simulink library "pwrsys"  (R2018a)
settings: Solver=VariableStepAuto  StartTime=0.0  StopTime=10.0  RelTol=1e-3
values from neighbouring files (symbols this model uses):
  Ts = Ts_c    (= 1e-07)    [PlantStateEquations_abc_Script.m]
undefined symbols (not defined in the file or in its folder): D1, Delta, DiscIntNeverNeededParam, ESS, f_LPF_noise, fn, fsw, grid, gt1, Iap, Kp, PCC, Refmax, Refmin, sim, SIMU, Sn, tctrl, Ti, Ts_control, Ts_PWM, Uabp, Uanp, WT, X, zeta
libraries: $bdroot x71, powerlib x59, powerlib_meascontrol x49, peTransforms x20, PhD_Library x1, sps_avr x1
(part 2 of 4)

== system pwrsys/Basic Blocks/PI_Kg_Kp_Ti_AntiWindup ==
  note: PI: Kg (Kp + 1/sTi)
  error : Inport
  DisableP : Inport  Port=2
  Ihold : Inport  Port=3
  force_int : Inport  Port=4
  force_val : Inport  Port=5
  Add1 : Sum
  Add9 : Sum
  Constant : Constant  Value=PI_max
  Constant1 : Constant  Value=PI_min
  Constant8 : Constant  Value=0
  Gain1 : Gain  Gain=Kp
  Gain7 : Gain  Gain=Kg
  Gain9 : Gain  Gain=1/Ti
  NotEqual : RelationalOperator  Operator=~=  OutDataTypeStr=boolean  RndMeth=Simplest
  Product : Product
  Relay : Relay  OnSwitchValue=0.6  OffSwitchValue=0.4  OnOutputValue=0  OffOutputValue=1
  Saturation1 : Saturate  UpperLimit=PI_max  LowerLimit=PI_min
  Switch : Switch  Criteria=u2 > Threshold
  digital_integrator : $bdroot/Basic Blocks/digital_integrator  Ts=Ts
  out : Outport
  Punlim : Outport  Port=2
  I : Outport  Port=3
  wires:
  NotEqual/1 -> [StopInt]
  Saturation1/1 -> out/1, NotEqual/2
  error/1 -> Gain7/1
  digital_integrator/1 -> I/1, Add9/2
  Add1/1 -> Switch/2
  Constant8/1 -> Switch/1
  Gain7/1 -> Gain1/1, Switch/3
  Switch/1 -> Gain9/1
  Add9/1 -> NotEqual/1, Saturation1/1
  Gain9/1 -> digital_integrator/1
  [StopInt] -> Add1/1
  Ihold/1 -> Add1/2
  Product/1 -> Punlim/1, Add9/1
  Gain1/1 -> Product/2
  DisableP/1 -> Relay/1
  Relay/1 -> Product/1
  force_val/1 -> digital_integrator/5
  force_int/1 -> digital_integrator/4
  Constant1/1 -> digital_integrator/3
  Constant/1 -> digital_integrator/2

== system pwrsys/Basic Blocks/PI_Kp_Ti_AntiWindup ==
  note: PI: Kp (s Ti + 1) / (s Ti)
  error : Inport
  Ihold : Inport  Port=2
  force_int : Inport  Port=3
  force_val : Inport  Port=4
  Add1 : Sum
  Add9 : Sum
  Constant : Constant  Value=PI_max
  Constant1 : Constant  Value=PI_min
  Constant8 : Constant  Value=0
  Gain7 : Gain  Gain=Kp
  Gain9 : Gain  Gain=1/Ti
  NotEqual : RelationalOperator  Operator=~=  OutDataTypeStr=boolean  RndMeth=Simplest
  Saturation1 : Saturate  UpperLimit=PI_max  LowerLimit=PI_min
  Switch : Switch  Criteria=u2 > Threshold
  digital_integrator : $bdroot/Basic Blocks/digital_integrator  Ts=Ts
  out : Outport
  Punlim : Outport  Port=2
  I : Outport  Port=3
  wires:
  NotEqual/1 -> [StopInt]
  Saturation1/1 -> out/1, NotEqual/2
  error/1 -> Gain7/1
  digital_integrator/1 -> I/1, Add9/2
  Add1/1 -> Switch/2
  Constant8/1 -> Switch/1
  Gain7/1 -> Switch/3, Punlim/1, Add9/1
  Switch/1 -> Gain9/1
  Add9/1 -> NotEqual/1, Saturation1/1
  Gain9/1 -> digital_integrator/1
  [StopInt] -> Add1/1
  Ihold/1 -> Add1/2
  Constant1/1 -> digital_integrator/3
  force_int/1 -> digital_integrator/4
  force_val/1 -> digital_integrator/5
  Constant/1 -> digital_integrator/2

== system pwrsys/Basic Blocks/PQVI ==
  note: Akagi 1984 for p and q
      | calc. without zero seq,
      | factor 3/2 compensates for
      | amplitude invariant
      | Clarke transformation
  valphabeta : Inport
  ialphabeta : Inport  Port=2
  Add3 : Sum  Inputs=+-
  Bus Creator : BusCreator  Inputs=4
  Demux1 : Demux  Outputs=2
  Demux4 : Demux  Outputs=2
  Dot Product : DotProduct  InputSameDT=on  OutDataTypeStr=Inherit: Inherit via internal rule
  Gain1 : Gain  Gain=3/2/Sn
  Gain2 : Gain  Gain=3/2/Sn
  Gain3 : Gain  Gain=1/Uanp
  Gain4 : Gain  Gain=1/Iap
  Hypot : Math  Operator=hypot  RndMeth=Zero  SaturateOnIntegerOverflow=on
  Hypot1 : Math  Operator=hypot  RndMeth=Zero  SaturateOnIntegerOverflow=on
  Product3 : Product
  Product4 : Product
  pqvi : Outport
  wires:
  Gain4/1 -> Bus Creator/4  "i"
  Gain1/1 -> Bus Creator/1  "p"
  Gain2/1 -> Bus Creator/2  "q"
  Product4/1 -> Add3/2
  Dot Product/1 -> Gain1/1  "p"
  Hypot1/1 -> Gain4/1  "i"
  Gain3/1 -> Bus Creator/3  "v"
  Demux1/2 -> Hypot1/2, Product4/2
  valphabeta/1 -> Demux4/1, Dot Product/1
  Demux1/1 -> Hypot1/1, Product3/2
  ialphabeta/1 -> Demux1/1, Dot Product/2
  Add3/1 -> Gain2/1  "q"
  Demux4/2 -> Hypot/2, Product3/1
  Product3/1 -> Add3/1
  Hypot/1 -> Gain3/1  "v"
  Demux4/1 -> Hypot/1, Product4/1
  Bus Creator/1 -> pqvi/1

== system pwrsys/Basic Blocks/digital_integrator ==
  x : Inport
  max : Inport  Port=2
  min : Inport  Port=3
  force_if=1 : Inport  Port=4
  force_value : Inport  Port=5
  Constant : Constant  Value=Ts
  MATLAB Function : MATLAB Function  TreatAsAtomicUnit=on  SystemSampleTime=Ts
      settings: RTWSystemCode=Inline
  y : Outport
  wires:
  x/1 -> MATLAB Function/1(x)
  MATLAB Function/1(y) -> y/1
  max/1 -> MATLAB Function/2(max)
  min/1 -> MATLAB Function/3(min)
  force_if=1/1 -> MATLAB Function/4(force)
  force_value/1 -> MATLAB Function/5(forceval)
  Constant/1 -> MATLAB Function/6(Ts)

== system pwrsys/Basic Blocks/digital_ramp_gen ==
  up_if>0 : Inport
  down_if>0 : Inport  Port=2
  rate_pu/s : Inport  Port=3
  max : Inport  Port=4
  min : Inport  Port=5
  force_if=1 : Inport  Port=6
  force_value : Inport  Port=7
  Constant : Constant  Value=Ts
  MATLAB Function : MATLAB Function  TreatAsAtomicUnit=on  SystemSampleTime=Ts
      settings: RTWSystemCode=Inline
  y : Outport
  wires:
  up_if>0/1 -> MATLAB Function/1(up)
  MATLAB Function/1(y) -> y/1
  max/1 -> MATLAB Function/4(max)
  min/1 -> MATLAB Function/5(min)
  force_if=1/1 -> MATLAB Function/6(force)
  force_value/1 -> MATLAB Function/7(forceval)
  Constant/1 -> MATLAB Function/8(Ts)
  down_if>0/1 -> MATLAB Function/2(down)
  rate_pu/s/1 -> MATLAB Function/3(rate)

== system pwrsys/Basic Blocks/pqui_Transd_DSC ==
  Vabc : Inport
  Iabc : Inport  Port=2
  w_pu : Inport  Port=3
  Clarke Transform{,1..3} (4 alike) : peTransforms/Clarke Transform  PowerInvariant=off
  Constant : Constant
  DSC Power 1 : $bdroot/Basic Blocks/DSC Power 
  DSC Power 2 : $bdroot/Basic Blocks/DSC Power 
  Data Type Conversion1 : DataTypeConversion  OutDataTypeStr=int16  RndMeth=Round  SaturateOnIntegerOverflow=on
  Divide : Product  Inputs=*/
  Gain2 : Gain  Gain=4*Ts*fn
  PQVI : $bdroot/Basic Blocks/PQVI  Sn=Sn  Uanp=Uanp  Iap=Iap
  PQVI_Neg : $bdroot/Basic Blocks/PQVI  Sn=Sn  Uanp=Uanp  Iap=Iap
  PQVI_Pos : $bdroot/Basic Blocks/PQVI  Sn=Sn  Uanp=Uanp  Iap=Iap
  Rate Transition1 : RateTransition  OutPortSampleTime=Ts
  Rate Transition2 : RateTransition  InitialCondition=1  OutPortSampleTime=Ts
  Rate Transition5 : RateTransition  OutPortSampleTime=Ts
  Saturation : Saturate  UpperLimit=inf  LowerLimit=0.000001
  Selector{1,4..6} (4 alike) : Selector  InputPortWidth=3  IndexOptions=Index vector (dialog)  Indices=[1 2]  OutputSizes=1
  Selector2 : Selector  InputPortWidth=3  IndexOptions=Index vector (dialog)  Indices=[1 3 2]  OutputSizes=1
  Selector3 : Selector  InputPortWidth=3  IndexOptions=Index vector (dialog)  Indices=[1 3 2]  OutputSizes=1
  pqvi : Outport
  pqvi+ : Outport  Port=2
  pqvi- : Outport  Port=3
  wires:
  Clarke Transform1/1 -> Selector1/1
  Vabc/1 -> Rate Transition1/1
  Clarke Transform/1 -> Selector5/1
  Iabc/1 -> Rate Transition5/1
  Rate Transition1/1 -> Selector2/1, Clarke Transform/1
  Rate Transition5/1 -> Selector3/1, Clarke Transform1/1
  Selector5/1 -> DSC Power 2/1, PQVI/1
  Selector1/1 -> DSC Power 2/2, PQVI/2
  PQVI/1 -> pqvi/1
  Data Type Conversion1/1 -> DSC Power 1/3, DSC Power 2/3
  DSC Power 2/1 -> PQVI_Pos/1
  DSC Power 2/2 -> PQVI_Pos/2
  PQVI_Pos/1 -> pqvi+/1
  Clarke Transform2/1 -> Selector6/1
  Clarke Transform3/1 -> Selector4/1
  Selector2/1 -> Clarke Transform2/1
  Selector3/1 -> Clarke Transform3/1
  Selector6/1 -> DSC Power 1/1
  Selector4/1 -> DSC Power 1/2
  PQVI_Neg/1 -> pqvi-/1
  DSC Power 1/2 -> PQVI_Neg/2
  DSC Power 1/1 -> PQVI_Neg/1
  Saturation/1 -> Divide/2
  Constant/1 -> Divide/1
  Rate Transition2/1 -> Gain2/1
  w_pu/1 -> Rate Transition2/1
  Gain2/1 -> Saturation/1
  Divide/1 -> Data Type Conversion1/1

== system pwrsys/Basic Blocks/pqui_Transd_NoZeroSeq ==
  note: Akagi 1984 for p and q
      | calc. without zero seq,
      | factor 3/2 compensates for
      | amplitude invariant
      | Clarke transformation
  Vabc : Inport
  Iabc : Inport  Port=2
  Add3 : Sum  Inputs=+-
  Clarke Transform : peTransforms/Clarke Transform  PowerInvariant=off
  Clarke Transform1 : peTransforms/Clarke Transform  PowerInvariant=off
  Demux1 : Demux  Outputs=2
  Demux4 : Demux  Outputs=2
  Dot Product : DotProduct  InputSameDT=on  OutDataTypeStr=Inherit: Inherit via internal rule
  Gain1 : Gain  Gain=3/2/Sn
  Gain2 : Gain  Gain=3/2/Sn
  Gain3 : Gain  Gain=1/Uanp
  Gain4 : Gain  Gain=1/Iap
  Hypot : Math  Operator=hypot  RndMeth=Zero  SaturateOnIntegerOverflow=on
  Hypot1 : Math  Operator=hypot  RndMeth=Zero  SaturateOnIntegerOverflow=on
  Product3 : Product
  Product4 : Product
  Selector1 : Selector  InputPortWidth=3  IndexOptions=Index vector (dialog)  Indices=[1 2]  OutputSizes=1
  Selector5 : Selector  InputPortWidth=3  IndexOptions=Index vector (dialog)  Indices=[1 2]  OutputSizes=1
  p : Outport
  q : Outport  Port=2
  v : Outport  Port=3
  i : Outport  Port=4
  wires:
  Clarke Transform1/1 -> Selector1/1
  Gain3/1 -> v/1  "v"
  Demux1/2 -> Hypot1/2, Product4/2
  Hypot1/1 -> Gain4/1  "i"
  Selector1/1 -> Demux1/1, Dot Product/2
  Selector5/1 -> Demux4/1, Dot Product/1
  Demux4/1 -> Hypot/1, Product4/1
  Hypot/1 -> Gain3/1  "v"
  Dot Product/1 -> Gain1/1  "p"
  Demux1/1 -> Hypot1/1, Product3/2
  Add3/1 -> Gain2/1  "q"
  Product4/1 -> Add3/2
  Demux4/2 -> Hypot/2, Product3/1
  Vabc/1 -> Clarke Transform/1
  Clarke Transform/1 -> Selector5/1
  Iabc/1 -> Clarke Transform1/1
  Product3/1 -> Add3/1
  Gain1/1 -> p/1  "p"
  Gain4/1 -> i/1  "i"
  Gain2/1 -> q/1  "q"

== system pwrsys/Basic Blocks/pqui_Transd_NoZeroSeq_Filter ==
  note: Akagi 1984 for p and q
      | calc. without zero seq,
      | factor 3/2 compensates for
      | amplitude invariant
      | Clarke transformation
  Vabc : Inport
  Iabc : Inport  Port=2
  Add3 : Sum  Inputs=+-
  Clarke Transform : peTransforms/Clarke Transform  PowerInvariant=off
  Clarke Transform1 : peTransforms/Clarke Transform  PowerInvariant=off
  Demux1 : Demux  Outputs=2
  Demux4 : Demux  Outputs=2
  Dot Product : DotProduct  InputSameDT=on  OutDataTypeStr=Inherit: Inherit via internal rule
  Gain1 : Gain  Gain=3/2/Sn
  Gain2 : Gain  Gain=3/2/Sn
  Gain3 : Gain  Gain=1/Uanp
  Gain4 : Gain  Gain=1/Iap
  Hypot : Math  Operator=hypot  RndMeth=Zero  SaturateOnIntegerOverflow=on
  Hypot1 : Math  Operator=hypot  RndMeth=Zero  SaturateOnIntegerOverflow=on
  Product3 : Product
  Product4 : Product
  Rate Transition1 : RateTransition  OutPortSampleTime=Ts
  Rate Transition2 : RateTransition  OutPortSampleTime=Ts
  Second-Order Filter1 : powerlib_meascontrol/Filters/Second-Order Filter  FilterType=Lowpass  Fo=fcutoutvi  Zeta=zeta  Ts=Ts  Initialize=off  Vac_Init="[0,  0,  60]"  Vdc_Init=0  PlotResponse=off  FreqRange=[0, 1000, 0.1]
      settings: SourceProductName=Simscape Power Systems  SourceProductBaseCode=PS
  Second-Order Filter2 : powerlib_meascontrol/Filters/Second-Order Filter  FilterType=Lowpass  Fo=fcutoutvi  Zeta=zeta  Ts=Ts  Initialize=off  Vac_Init="[0,  0,  60]"  Vdc_Init=0  PlotResponse=off  FreqRange=[0, 1000, 0.1]
      settings: SourceProductName=Simscape Power Systems  SourceProductBaseCode=PS
  Second-Order Filter{3,5..6,8} (4 alike) : powerlib_meascontrol/Filters/Second-Order Filter  FilterType=Bandstop (Notch)  Fo=fn  Zeta=zeta  Ts=Ts  Initialize=off  Vac_Init="[0,  0,  60]"  Vdc_Init=0  PlotResponse=off  FreqRange=[0, 1000, 0.1]
      settings: SourceProductName=Simscape Power Systems  SourceProductBaseCode=PS
  Second-Order Filter4 : powerlib_meascontrol/Filters/Second-Order Filter  FilterType=Lowpass  Fo=fcutoutpq  Zeta=zeta  Ts=Ts  Initialize=off  Vac_Init="[0,  0,  60]"  Vdc_Init=0  PlotResponse=off  FreqRange=[0, 1000, 0.1]
      settings: SourceProductName=Simscape Power Systems  SourceProductBaseCode=PS
  Second-Order Filter7 : powerlib_meascontrol/Filters/Second-Order Filter  FilterType=Lowpass  Fo=fcutoutpq  Zeta=zeta  Ts=Ts  Initialize=off  Vac_Init="[0,  0,  60]"  Vdc_Init=0  PlotResponse=off  FreqRange=[0, 1000, 0.1]
      settings: SourceProductName=Simscape Power Systems  SourceProductBaseCode=PS
  Selector1 : Selector  InputPortWidth=3  IndexOptions=Index vector (dialog)  Indices=[1 2]  OutputSizes=1
  Selector5 : Selector  InputPortWidth=3  IndexOptions=Index vector (dialog)  Indices=[1 2]  OutputSizes=1
  p : Outport
  q : Outport  Port=2
  v : Outport  Port=3
  i : Outport  Port=4
  wires:
  Clarke Transform1/1 -> Selector1/1
  Gain3/1 -> Second-Order Filter2/1  "v"
  Demux1/2 -> Hypot1/2, Product4/2
  Hypot1/1 -> Gain4/1  "i"
  Selector1/1 -> Demux1/1, Dot Product/2
  Selector5/1 -> Demux4/1, Dot Product/1
  Demux4/1 -> Hypot/1, Product4/1
  Hypot/1 -> Gain3/1  "v"
  Iabc/1 -> Rate Transition2/1
  Dot Product/1 -> Gain1/1  "p"
  Demux1/1 -> Hypot1/1, Product3/2
  Add3/1 -> Gain2/1  "q"
  Vabc/1 -> Rate Transition1/1
  Product4/1 -> Add3/2
  Demux4/2 -> Hypot/2, Product3/1
  Rate Transition1/1 -> Clarke Transform/1
  Clarke Transform/1 -> Selector5/1
  Rate Transition2/1 -> Clarke Transform1/1
  Product3/1 -> Add3/1
  Gain1/1 -> Second-Order Filter7/1  "p"
  Gain4/1 -> Second-Order Filter1/1  "i"
  Gain2/1 -> Second-Order Filter4/1  "q"
  Second-Order Filter2/1 -> Second-Order Filter5/1
  Second-Order Filter5/1 -> v/1
  Second-Order Filter1/1 -> Second-Order Filter3/1
  Second-Order Filter3/1 -> i/1
  Second-Order Filter4/1 -> Second-Order Filter6/1
  Second-Order Filter6/1 -> q/1
  Second-Order Filter8/1 -> p/1
  Second-Order Filter7/1 -> Second-Order Filter8/1

== system pwrsys/PLLs/PLL ==
  vabc : Inport
  PLL (3ph) : powerlib_meascontrol/PLL/PLL (3ph)  Fmin=0.8*fn  Par_Init=[PLL_ini, fn]  ParK=[Kp_pll, Ki_pll, Kd_pll]  TcD=1e-4  MaxRateChangeFreq=fn/5  FilterCutOffFreq=fn/2  Ts=Ts  AGC=on
  Rate Transition1 : RateTransition  OutPortSampleTime=Ts
  Rtot_pu1 : Gain  Gain=-1  SaturateOnIntegerOverflow=on  OutDataTypeStr=Inherit: Same as input  ParamDataTypeStr=Inherit: Same as input
  Rtot_pu3 : Gain  Gain=1/fn  SaturateOnIntegerOverflow=on  OutDataTypeStr=Inherit: Same as input  ParamDataTypeStr=Inherit: Same as input
  f_pu : Outport
  wt : Outport  Port=2
  minus_wt : Outport  Port=3
  wires:
  Rtot_pu3/1 -> f_pu/1
  vabc/1 -> Rate Transition1/1
  Rate Transition1/1 -> PLL (3ph)/1
  PLL (3ph)/2 -> Rtot_pu1/1, wt/1
  PLL (3ph)/1 -> Rtot_pu3/1
  Rtot_pu1/1 -> minus_wt/1

== system pwrsys/PLLs/PLL 3-phase abc ==
  Vabc : Inport
  120deg : Constant  Value=2/3*pi
  Anti-windup : RelationalOperator  Operator=~=  OutDataTypeStr=boolean  RndMeth=Simplest
  Derivative : Gain  Gain=Kd/Tr
  Discrete-Time Integrator : DiscreteIntegrator  gainval=1/Tr  SampleTime=-1  LimitOutput=on  UpperSaturationLimit=2*pi*fdev  LowerSaturationLimit=-2*pi*fdev  ICPrevOutput=DiscIntNeverNeededParam  ICPrevScaledInput=DiscIntNeverNeededParam
  Dot Product : DotProduct  InputSameDT=on  OutDataTypeStr=Inherit: Inherit via internal rule
  Integrator : Integrator  InitialCondition=wt0  UpperSaturationLimit=1  LowerSaturationLimit=-1  ZeroCross=off
  Mux : Mux  Inputs=2
  Mux1 : Mux  Inputs=3
  PI controller with Hold : $bdroot/Basic Blocks/PI controller  with Hold  Kp=Kp  Ki=Ki  Max=2*pi*fdev  Min=-2*pi*fdev  x0=0  Ts=Ts
  Saturation : Saturate  UpperLimit=2*pi*fdev  LowerLimit=-2*pi*fdev
  Second-Order Filter : powerlib_meascontrol/Filters/Second-Order Filter  FilterType=Lowpass  Fo=wn  Zeta=zeta  Ts=0  Initialize=on  Vac_Init="[0,  0,  60]"  Vdc_Init=2*pi*fnom  PlotResponse=off  FreqRange=[0, 500, 1]
      settings: SourceProductName=Simscape Power Systems  SourceProductBaseCode=PS
  Sum1 : Sum
  Sum2 : Sum  Inputs=+-
  Sum3 : Sum
  Sum4 : Sum  Inputs=+-
  Sum6 : Sum  Inputs=-+
  Trigonometric Function : Trigonometry  Operator=sincos  ApproximationMethod=CORDIC
  Trigonometric Function1 : Trigonometry  ApproximationMethod=CORDIC
  Wrap to pi : MATLABFcn  MATLABFcn=wrapToPi
  w rated : Constant  Value=2*pi*fnom
  w : Outport
  wt : Outport  Port=2
  scwt : Outport  Port=3
  wires:
  Discrete-Time Integrator/1 -> Sum6/1
  Sum6/1 -> Discrete-Time Integrator/1, Sum2/2  "d"
  Derivative/1 -> Sum6/2
  Saturation/1 -> Sum1/1, Anti-windup/2  "dw"
  w rated/1 -> Sum1/2
  Sum1/1 -> Second-Order Filter/1, Integrator/1  "w"
  Integrator/1 -> Wrap to pi/1  "wt"
  Vabc/1 -> Dot Product/1
  PI controller with Hold/1 -> Sum2/1  "pi"
  Sum2/1 -> Anti-windup/1, Saturation/1
  Wrap to pi/1 -> Mux1/1, Trigonometric Function/1, Sum4/1, Sum3/1, wt/1  "wtWrap"
  Trigonometric Function/1 -> Mux/1
  Trigonometric Function/2 -> Mux/2
  Mux/1 -> scwt/1
  120deg/1 -> Sum4/2, Sum3/2
  Sum4/1 -> Mux1/2
  Sum3/1 -> Mux1/3
  Mux1/1 -> Trigonometric Function1/1
  Trigonometric Function1/1 -> Dot Product/2
  Second-Order Filter/1 -> w/1
  Dot Product/1 -> Derivative/1, PI controller with Hold/2
  Anti-windup/1 -> PI controller with Hold/1

== system pwrsys/PLLs/PLL_pu ==
  vabc : Inport
  PLL (3ph) : powerlib_meascontrol/PLL/PLL (3ph)  Fmin=0.8*fn  Par_Init=[PLL_ini, fn]  ParK=[Kp_pll, Ki_pll, Kd_pll]  TcD=1e-4  MaxRateChangeFreq=fn/5  FilterCutOffFreq=fn/2  Ts=Ts  AGC=on
  Rate Transition1 : RateTransition  OutPortSampleTime=Ts
  Rtot_pu3 : Gain  Gain=1/fn  SaturateOnIntegerOverflow=on  OutDataTypeStr=Inherit: Same as input  ParamDataTypeStr=Inherit: Same as input
  wt : Outport
  f_pu : Outport  Port=2
  wires:
  Rtot_pu3/1 -> f_pu/1
  vabc/1 -> Rate Transition1/1
  Rate Transition1/1 -> PLL (3ph)/1
  PLL (3ph)/2 -> wt/1
  PLL (3ph)/1 -> Rtot_pu3/1

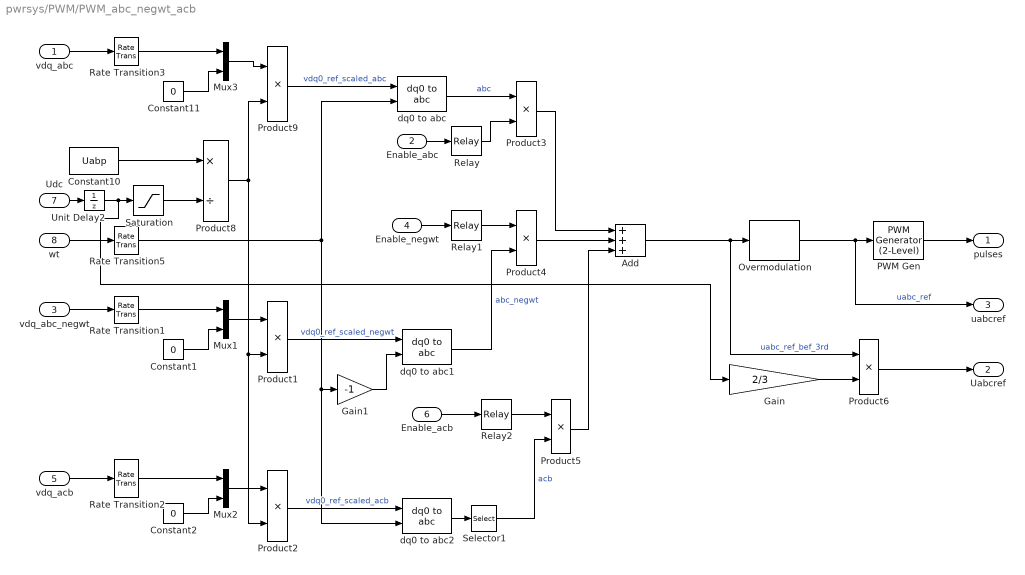
== system pwrsys/PWM/PWM_abc_negwt_acb ==
  vdq_abc : Inport
  Enable_abc : Inport  Port=2
  vdq_abc_negwt : Inport  Port=3
  Enable_negwt : Inport  Port=4
  vdq_acb : Inport  Port=5
  Enable_acb : Inport  Port=6
  Udc : Inport  Port=7
  wt : Inport  Port=8
  Add : Sum  Inputs=+++
  Constant1 : Constant  Value=0
  Constant10 : Constant  Value=Uabp
  Constant11 : Constant  Value=0
  Constant2 : Constant  Value=0
  Gain : Gain  Gain=2/3
  Gain1 : Gain  Gain=-1
  Mux1 : Mux  Inputs=[2 1]
  Mux2 : Mux  Inputs=[2 1]
  Mux3 : Mux  Inputs=[2 1]
  Overmodulation : powerlib_meascontrol/Pulse & Signal Generators/Overmodulation  OverModType=Third harmonic
      settings: SourceProductName=Simscape Power Systems  SourceProductBaseCode=PS
  PWM Gen : powerlib_meascontrol/Pulse & Signal Generators/PWM Generator (2-Level)  ModulatorType=Three-phase bridge (6 pulses)  ModulatorMode=Unsynchronized  Fc=fsw  Pc=PWM_Ini_Phase  nF=27  MinMax="[ -1  1 ]"  SamplingTechnique=Asymmetrical regular (double edge)  ModulatingSignals=off  m=0.8  Freq=60  Phase=0  Ts=Ts  ShowCarrierOutport=off
      settings: SourceProductName=Simscape Power Systems
  Product{1..6,9} (7 alike) : Product  Inputs=**
  Product8 : Product  Inputs=*/
  Rate Transition{1..3,5} (4 alike) : RateTransition  OutPortSampleTime=Ts
  Relay : Relay  OnSwitchValue=0.6  OffSwitchValue=0.4
  Relay1 : Relay  OnSwitchValue=0.6  OffSwitchValue=0.4
  Relay2 : Relay  OnSwitchValue=0.6  OffSwitchValue=0.4
  Saturation : Saturate  UpperLimit=10*Uabp  LowerLimit=0.001*Uabp
  Selector1 : Selector  InputPortWidth=3  IndexOptions=Index vector (dialog)  Indices=[1 3 2]  OutputSizes=1
  Unit Delay2 : UnitDelay  InitialCondition=Uabp  SampleTime=Ts
  dq0 to abc : powerlib_meascontrol/Transformations/dq0 to abc  Alignment=90 degrees behind phase A axis
  dq0 to abc1 : powerlib_meascontrol/Transformations/dq0 to abc  Alignment=90 degrees behind phase A axis
  dq0 to abc2 : powerlib_meascontrol/Transformations/dq0 to abc  Alignment=90 degrees behind phase A axis
  pulses : Outport
  Uabcref : Outport  Port=2
  uabcref : Outport  Port=3
  wires:
  dq0 to abc1/1 -> Product4/2  "abc_negwt"
  Gain1/1 -> dq0 to abc1/2
  Product1/1 -> dq0 to abc1/1  "vdq0_ref_scaled_negwt"
  vdq_abc_negwt/1 -> Rate Transition1/1
  Constant1/1 -> Mux1/2
  Mux1/1 -> Product1/1
  Rate Transition1/1 -> Mux1/1
  Product6/1 -> Uabcref/1
  vdq_abc/1 -> Rate Transition3/1
  PWM Gen/1 -> pulses/1
  Udc/1 -> Unit Delay2/1
  Overmodulation/1 -> uabcref/1, PWM Gen/1  "uabc_ref"
  Constant10/1 -> Product8/1
  wt/1 -> Rate Transition5/1
  Rate Transition3/1 -> Mux3/1
  Mux3/1 -> Product9/1
  Unit Delay2/1 -> Gain/1, Saturation/1
  Product9/1 -> dq0 to abc/1  "vdq0_ref_scaled_abc"
  Rate Transition5/1 -> dq0 to abc/2, dq0 to abc2/2, Gain1/1
  Constant11/1 -> Mux3/2
  dq0 to abc/1 -> Product3/1  "abc"
  Enable_abc/1 -> Relay/1
  Enable_negwt/1 -> Relay1/1
  Add/1 -> Product6/1, Overmodulation/1  "uabc_ref_bef_3rd"
  Saturation/1 -> Product8/2
  Product8/1 -> Product2/2, Product1/2, Product9/2
  Rate Transition2/1 -> Mux2/1
  vdq_acb/1 -> Rate Transition2/1
  Enable_acb/1 -> Relay2/1
  Mux2/1 -> Product2/1
  Constant2/1 -> Mux2/2
  Product2/1 -> dq0 to abc2/1  "vdq0_ref_scaled_acb"
  dq0 to abc2/1 -> Selector1/1
  Selector1/1 -> Product5/2  "acb"
  Relay/1 -> Product3/2
  Product3/1 -> Add/1
  Product4/1 -> Add/2
  Relay1/1 -> Product4/1
  Relay2/1 -> Product5/1
  Product5/1 -> Add/3
  Gain/1 -> Product6/2

== system pwrsys/PWM/PWM_single_dual ==
  vdq_single : Inport
  Enable_single : Inport  Port=2
  vdq_dual_pos : Inport  Port=3
  vdq_dual_neg : Inport  Port=4
  Enable_dual : Inport  Port=5
  Udc : Inport  Port=6
  wt : Inport  Port=7
  Add : Sum  Inputs=+++
  Constant1 : Constant  Value=0
  Constant10 : Constant  Value=Uabp
  Constant11 : Constant  Value=0
  Constant2 : Constant  Value=0
  Gain : Gain  Gain=2/3
  Mux1 : Mux  Inputs=[2 1]
  Mux2 : Mux  Inputs=[2 1]
  Mux3 : Mux  Inputs=[2 1]
  Overmodulation : powerlib_meascontrol/Pulse & Signal Generators/Overmodulation  OverModType=Third harmonic
      settings: SourceProductName=Simscape Power Systems  SourceProductBaseCode=PS
  PWM Gen : powerlib_meascontrol/Pulse & Signal Generators/PWM Generator (2-Level)  ModulatorType=Three-phase bridge (6 pulses)  ModulatorMode=Unsynchronized  Fc=fsw  Pc=PWM_Ini_Phase  nF=27  MinMax="[ -1  1 ]"  SamplingTechnique=Asymmetrical regular (double edge)  ModulatingSignals=off  m=0.8  Freq=60  Phase=0  Ts=Ts  ShowCarrierOutport=off
      settings: SourceProductName=Simscape Power Systems
  Product{1..6,9} (7 alike) : Product  Inputs=**
  Product8 : Product  Inputs=*/
  Rate Transition{1..3,5} (4 alike) : RateTransition  OutPortSampleTime=Ts
  Relay : Relay  OnSwitchValue=0.6  OffSwitchValue=0.4
  Relay1 : Relay  OnSwitchValue=0.6  OffSwitchValue=0.4
  Saturation : Saturate  UpperLimit=10*Uabp  LowerLimit=0.001*Uabp
  Selector1 : Selector  InputPortWidth=3  IndexOptions=Index vector (dialog)  Indices=[1 3 2]  OutputSizes=1
  Unit Delay2 : UnitDelay  InitialCondition=Uabp  SampleTime=Ts
  dq0 to abc : powerlib_meascontrol/Transformations/dq0 to abc  Alignment=90 degrees behind phase A axis
  dq0 to abc1 : powerlib_meascontrol/Transformations/dq0 to abc  Alignment=90 degrees behind phase A axis
  dq0 to abc2 : powerlib_meascontrol/Transformations/dq0 to abc  Alignment=90 degrees behind phase A axis
  pulses : Outport
  Uabcref : Outport  Port=2
  uabcref : Outport  Port=3
  wires:
  dq0 to abc1/1 -> Product4/2  "abc_ref_dual_pos"
  Rate Transition5/1 -> dq0 to abc/2, dq0 to abc1/2, dq0 to abc2/2
  Product1/1 -> dq0 to abc1/1  "vdq0_ref_scaled_dual_pos"
  vdq_dual_pos/1 -> Rate Transition1/1
  Constant1/1 -> Mux1/2
  Mux1/1 -> Product1/1
  Rate Transition1/1 -> Mux1/1
  Product6/1 -> Uabcref/1
  vdq_single/1 -> Rate Transition3/1
  PWM Gen/1 -> pulses/1
  Udc/1 -> Unit Delay2/1
  Overmodulation/1 -> uabcref/1, PWM Gen/1  "uabc_ref"
  Constant10/1 -> Product8/1
  wt/1 -> Rate Transition5/1
  Rate Transition3/1 -> Mux3/1
  Mux3/1 -> Product9/1
  Unit Delay2/1 -> Gain/1, Saturation/1
  Product9/1 -> dq0 to abc/1  "vdq0_ref_scaled_single"
  Constant11/1 -> Mux3/2
  dq0 to abc/1 -> Product3/1  "abc_ref_single"
  Enable_single/1 -> Relay/1
  Enable_dual/1 -> Relay1/1
  Add/1 -> Product6/1, Overmodulation/1  "uabc_ref_bef_3rd"
  Saturation/1 -> Product8/2
  Product8/1 -> Product2/2, Product1/2, Product9/2
  Rate Transition2/1 -> Mux2/1
  vdq_dual_neg/1 -> Rate Transition2/1
  Mux2/1 -> Product2/1
  Constant2/1 -> Mux2/2
  Product2/1 -> dq0 to abc2/1  "vdq0_ref_scaled_dual_neg"
  dq0 to abc2/1 -> Selector1/1
  Selector1/1 -> Product5/2  "abc_ref_dual_neg"
  Relay/1 -> Product3/2
  Product3/1 -> Add/1
  Product4/1 -> Add/2
  Relay1/1 -> Product5/1, Product4/1
  Product5/1 -> Add/3
  Gain/1 -> Product6/2

== system pwrsys/Power Theories/Instantaneous Power xyz ==
  Vxyz : Inport
  Ixyz : Inport  Port=2
  Constant1 : Constant  Value=[a 0 0; 0 a 0; 0 0 b]
  Cross product terms : Product  RndMeth=Zero
  Demux2 : Demux  Outputs=2
  Dot Product : DotProduct  InputSameDT=on  OutDataTypeStr=Inherit: Inherit via internal rule
  Dot Product1 : DotProduct  InputSameDT=on  OutDataTypeStr=Inherit: Inherit via internal rule
  I elements : Selector  InputPortWidth=3  IndexOptions=Index vector (dialog)  Indices=[3 1 2 2 3 1]  OutputSizes=1
  P0 mult : Product  RndMeth=Zero
  Product3 : Product  Multiplication=Matrix(*)
  Q calc : Sum  Inputs=+-
  Sqrt : Sqrt  SaturateOnIntegerOverflow=on
  V elements : Selector  InputPortWidth=3  IndexOptions=Index vector (dialog)  Indices=[2 3 1 3 1 2]  OutputSizes=1
  i0 : Selector  InputPortWidth=3  IndexOptions=Index vector (dialog)  Indices=[3]  OutputSizes=1
  v0 : Selector  InputPortWidth=3  IndexOptions=Index vector (dialog)  Indices=[3]  OutputSizes=1
  P : Outport
  P0 : Outport  Port=2
  Qmat : Outport  Port=3
  Qnorm : Outport  Port=4
  wires:
  Dot Product/1 -> P/1  "P"
  Q calc/1 -> Qmat/1, Dot Product1/2, Dot Product1/1  "Qmat"
  Constant1/1 -> Product3/1
  Product3/1 -> V elements/1, v0/1, Dot Product/1
  Demux2/1 -> Q calc/1
  I elements/1 -> Cross product terms/2
  Vxyz/1 -> Product3/2
  Demux2/2 -> Q calc/2
  Ixyz/1 -> I elements/1, i0/1, Dot Product/2
  V elements/1 -> Cross product terms/1
  Cross product terms/1 -> Demux2/1
  v0/1 -> P0 mult/1
  i0/1 -> P0 mult/2
  P0 mult/1 -> P0/1  "P0"
  Dot Product1/1 -> Sqrt/1
  Sqrt/1 -> Qnorm/1  "Qnorm"

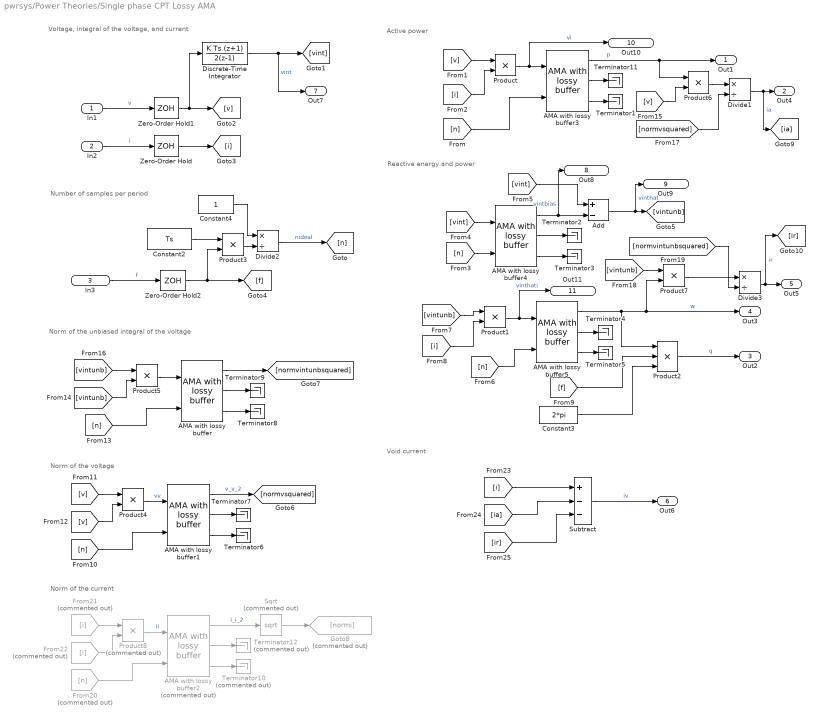
== system pwrsys/Power Theories/Single phase CPT Lossy AMA ==
  note: Voltage, integral of the voltage, and current
  note: Number of samples per period
  note: Norm of the unbiased integral of the voltage
  note: Norm of the voltage
  note: Active power
  note: Reactive energy and power
  note: Norm of the current
  note: Void current
  In1 : Inport
  In2 : Inport  Port=2
  In3 : Inport  Port=3
  AMA with lossy buffer{,1,3..5} (5 alike) : $bdroot/Adaptive Moving Averages/AMA with lossy buffer  NbSize=NbSize  Ts=Ts
  AMA with lossy buffer2 : $bdroot/Adaptive Moving Averages/AMA with lossy buffer  Commented=on  NbSize=NbSize  Ts=Ts
  Add : Sum  Inputs=+-
  Constant2 : Constant  Value=Ts
  Constant3 : Constant  Value=2*pi
  Constant4 : Constant
  Discrete-Time Integrator : DiscreteIntegrator  IntegratorMethod=Integration: Trapezoidal  SampleTime=Ts  ICPrevOutput=DiscIntNeverNeededParam  ICPrevScaledInput=DiscIntNeverNeededParam
  Divide1 : Product  Inputs=*/
  Divide2 : Product  Inputs=*/
  Divide3 : Product  Inputs=*/
  From20 : From  Commented=on  GotoTag=n
  From21 : From  Commented=on  GotoTag=i
  From22 : From  Commented=on  GotoTag=i
  Goto8 : Goto  Commented=on  GotoTag=normi
  Product{,1,3..7} (7 alike) : Product
  Product2 : Product  Inputs=3
  Product8 : Product  Commented=on
  Sqrt : Sqrt  Commented=on  SaturateOnIntegerOverflow=on
  Subtract : Sum  Inputs=+--
  Terminator{1..9,11} (10 alike) : Terminator
  Terminator10 : Terminator  Commented=on
  Terminator12 : Terminator  Commented=on
  Zero-Order Hold : ZeroOrderHold  SampleTime=Ts
  Zero-Order Hold1 : ZeroOrderHold  SampleTime=Ts
  Zero-Order Hold2 : ZeroOrderHold  SampleTime=Ts
  Out1 : Outport
  Out4 : Outport  Port=2
  Out2 : Outport  Port=3
  Out3 : Outport  Port=4
  Out5 : Outport  Port=5
  Out6 : Outport  Port=6
  Out7 : Outport  Port=7
  Out8 : Outport  Port=8
  Out9 : Outport  Port=9
  Out10 : Outport  Port=10
  Out11 : Outport  Port=11
  wires:
  [n] -> AMA with lossy buffer3/2
  AMA with lossy buffer3/2 -> Terminator11/1
  AMA with lossy buffer3/3 -> Terminator1/1
  Product1/1 -> Out11/1, AMA with lossy buffer5/1  "vinthati"
  AMA with lossy buffer4/1 -> Out8/1, Add/2  "vintbias"
  AMA with lossy buffer4/2 -> Terminator2/1
  [n] -> AMA with lossy buffer4/2
  AMA with lossy buffer5/3 -> Terminator5/1
  AMA with lossy buffer4/3 -> Terminator3/1
  [n] -> AMA with lossy buffer5/2
  AMA with lossy buffer5/1 -> Product7/2, Out3/1, Product2/1  "w"
  [i] -> Product/2
  In1/1 -> Zero-Order Hold1/1  "v"
  In2/1 -> Zero-Order Hold/1  "i"
  [vint] -> Add/1
  Constant4/1 -> Divide2/1
  Divide2/1 -> [n]  "nideal"
  Product3/1 -> Divide2/2
  [v] -> Product/1
  Constant2/1 -> Product3/1
  AMA with lossy buffer5/2 -> Terminator4/1
  [f] -> Product2/2
  Constant3/1 -> Product2/3
  [i] -> Product1/2
  [vint] -> AMA with lossy buffer4/1
  Zero-Order Hold1/1 -> [v], Discrete-Time Integrator/1
  AMA with lossy buffer3/1 -> Product6/1, Out1/1  "p"
  [vintunb] -> Product1/1
  In3/1 -> Zero-Order Hold2/1  "f"
  Product/1 -> Out10/1, AMA with lossy buffer3/1  "vi"
  Zero-Order Hold2/1 -> Product3/2, [f]
  Zero-Order Hold/1 -> [i]
  Product2/1 -> Out2/1  "q"
  Discrete-Time Integrator/1 -> Out7/1, [vint]  "vint"
  Add/1 -> Out9/1, [vintunb]  "vinthat"
  AMA with lossy buffer1/3 -> Terminator6/1
  AMA with lossy buffer1/2 -> Terminator7/1
  AMA with lossy buffer1/1 -> [normvsquared]  "v_v_2"
  [v] -> Product4/1
  [n] -> AMA with lossy buffer1/2
  Product4/1 -> AMA with lossy buffer1/1  "vv"
  [v] -> Product4/2
  [n] -> AMA with lossy buffer/2
  AMA with lossy buffer/2 -> Terminator9/1
  AMA with lossy buffer/1 -> [normvintunbsquared]
  [vintunb] -> Product5/1
  Product5/1 -> AMA with lossy buffer/1
  AMA with lossy buffer/3 -> Terminator8/1
  [vintunb] -> Product5/2
  [v] -> Product6/2
  Product6/1 -> Divide1/1
  [normvsquared] -> Divide1/2
  Divide1/1 -> [ia], Out4/1  "ia"
  [vintunb] -> Product7/1
  Product7/1 -> Divide3/1
  [normvintunbsquared] -> Divide3/2
  Divide3/1 -> [ir], Out5/1  "ir"
  From20/1 -> AMA with lossy buffer2/2
  AMA with lossy buffer2/2 -> Terminator12/1
  AMA with lossy buffer2/1 -> Sqrt/1  "i_i_2"
  From21/1 -> Product8/1
  Product8/1 -> AMA with lossy buffer2/1  "ii"
  AMA with lossy buffer2/3 -> Terminator10/1
  From22/1 -> Product8/2
  Sqrt/1 -> Goto8/1
  [i] -> Subtract/1
  [ia] -> Subtract/2
  [ir] -> Subtract/3
  Subtract/1 -> Out6/1  "iv"

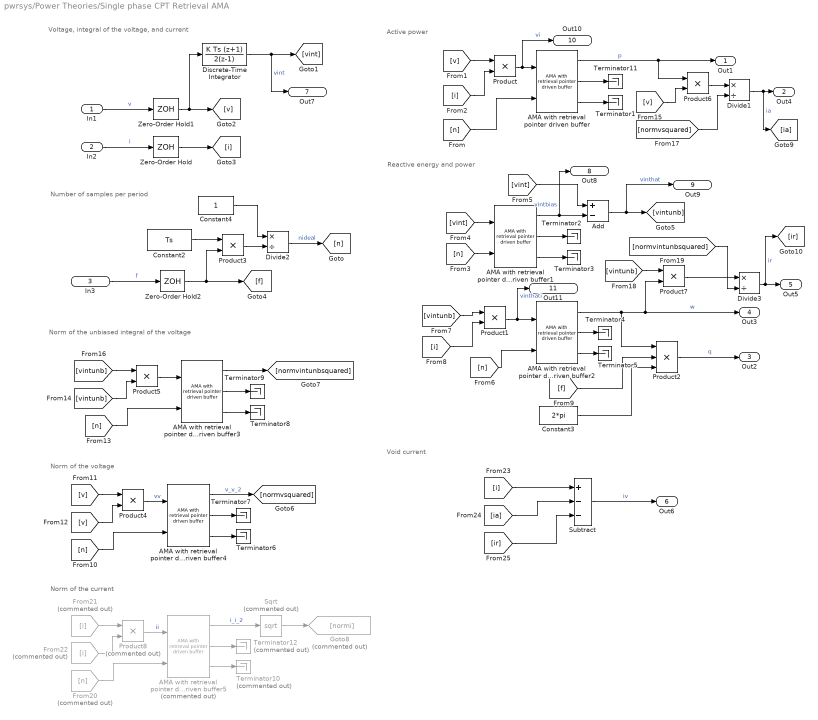
== system pwrsys/Power Theories/Single phase CPT Retrieval AMA ==
  note: Norm of the voltage
  note: Void current
  note: Active power
  note: Norm of the current
  note: Number of samples per period
  note: Norm of the unbiased integral of the voltage
  note: Reactive energy and power
  note: Voltage, integral of the voltage, and current
  In1 : Inport
  In2 : Inport  Port=2
  In3 : Inport  Port=3
  AMA with retrieval pointer driven buffer{,1..4} (5 alike) : $bdroot/Adaptive Moving Averages/AMA with retrieval pointer driven buffer  NbSize=NbSize  Ts=Ts
  AMA with retrieval pointer driven buffer5 : $bdroot/Adaptive Moving Averages/AMA with retrieval pointer driven buffer  Commented=on  NbSize=NbSize  Ts=Ts
  Add : Sum  Inputs=+-
  Constant2 : Constant  Value=Ts
  Constant3 : Constant  Value=2*pi
  Constant4 : Constant
  Discrete-Time Integrator : DiscreteIntegrator  IntegratorMethod=Integration: Trapezoidal  SampleTime=Ts  ICPrevOutput=DiscIntNeverNeededParam  ICPrevScaledInput=DiscIntNeverNeededParam
  Divide1 : Product  Inputs=*/
  Divide2 : Product  Inputs=*/
  Divide3 : Product  Inputs=*/
  From20 : From  Commented=on  GotoTag=n
  From21 : From  Commented=on  GotoTag=i
  From22 : From  Commented=on  GotoTag=i
  Goto8 : Goto  Commented=on  GotoTag=normi
  Product{,1,3..7} (7 alike) : Product
  Product2 : Product  Inputs=3
  Product8 : Product  Commented=on
  Sqrt : Sqrt  Commented=on  SaturateOnIntegerOverflow=on
  Subtract : Sum  Inputs=+--
  Terminator{1..9,11} (10 alike) : Terminator
  Terminator10 : Terminator  Commented=on
  Terminator12 : Terminator  Commented=on
  Zero-Order Hold : ZeroOrderHold  SampleTime=Ts
  Zero-Order Hold1 : ZeroOrderHold  SampleTime=Ts
  Zero-Order Hold2 : ZeroOrderHold  SampleTime=Ts
  Out1 : Outport
  Out4 : Outport  Port=2
  Out2 : Outport  Port=3
  Out3 : Outport  Port=4
  Out5 : Outport  Port=5
  Out6 : Outport  Port=6
  Out7 : Outport  Port=7
  Out8 : Outport  Port=8
  Out9 : Outport  Port=9
  Out10 : Outport  Port=10
  Out11 : Outport  Port=11
  wires:
  AMA with retrieval pointer driven buffer2/1 -> Product7/2, Out3/1, Product2/1  "w"
  [n] -> AMA with retrieval pointer driven buffer2/2
  [n] -> AMA with retrieval pointer driven buffer1/2
  [i] -> Subtract/1
  AMA with retrieval pointer driven buffer2/3 -> Terminator5/1
  AMA with retrieval pointer driven buffer/2 -> Terminator11/1
  AMA with retrieval pointer driven buffer/1 -> Product6/1, Out1/1  "p"
  Product4/1 -> AMA with retrieval pointer driven buffer4/1  "vv"
  [ia] -> Subtract/2
  [vintunb] -> Product5/1
  Divide3/1 -> [ir], Out5/1  "ir"
  From22/1 -> Product8/2
  Product8/1 -> AMA with retrieval pointer driven buffer5/1  "ii"
  AMA with retrieval pointer driven buffer5/3 -> Terminator10/1
  From21/1 -> Product8/1
  Divide1/1 -> [ia], Out4/1  "ia"
  [normvintunbsquared] -> Divide3/2
  Product7/1 -> Divide3/1
  [n] -> AMA with retrieval pointer driven buffer4/2
  Sqrt/1 -> Goto8/1
  [vintunb] -> Product7/1
  Product1/1 -> Out11/1, AMA with retrieval pointer driven buffer2/1  "vinthati"
  [v] -> Product6/2
  AMA with retrieval pointer driven buffer3/1 -> [normvintunbsquared]
  [normvsquared] -> Divide1/2
  AMA with retrieval pointer driven buffer3/2 -> Terminator9/1
  AMA with retrieval pointer driven buffer2/2 -> Terminator4/1
  AMA with retrieval pointer driven buffer4/1 -> [normvsquared]  "v_v_2"
  [n] -> AMA with retrieval pointer driven buffer3/2
  AMA with retrieval pointer driven buffer4/2 -> Terminator7/1
  Discrete-Time Integrator/1 -> Out7/1, [vint]  "vint"
  Zero-Order Hold/1 -> [i]
  In3/1 -> Zero-Order Hold2/1  "f"
  AMA with retrieval pointer driven buffer/3 -> Terminator1/1
  Zero-Order Hold1/1 -> [v], Discrete-Time Integrator/1
  [vintunb] -> Product1/1
  [i] -> Product1/2
  Constant3/1 -> Product2/3
  [f] -> Product2/2
  [vint] -> Add/1
  [ir] -> Subtract/3
  Constant2/1 -> Product3/1
  Product3/1 -> Divide2/2
  Divide2/1 -> [n]  "nideal"
  [v] -> Product/1
  Zero-Order Hold2/1 -> Product3/2, [f]
  [i] -> Product/2
  In2/1 -> Zero-Order Hold/1  "i"
  In1/1 -> Zero-Order Hold1/1  "v"
  AMA with retrieval pointer driven buffer3/3 -> Terminator8/1
  From20/1 -> AMA with retrieval pointer driven buffer5/2
  Product5/1 -> AMA with retrieval pointer driven buffer3/1
  [n] -> AMA with retrieval pointer driven buffer/2
  [v] -> Product4/1
  [vint] -> AMA with retrieval pointer driven buffer1/1
  AMA with retrieval pointer driven buffer1/2 -> Terminator2/1
  Subtract/1 -> Out6/1  "iv"
  AMA with retrieval pointer driven buffer4/3 -> Terminator6/1
  Product6/1 -> Divide1/1
  AMA with retrieval pointer driven buffer5/1 -> Sqrt/1  "i_i_2"
  Add/1 -> Out9/1, [vintunb]  "vinthat"
  Product/1 -> Out10/1, AMA with retrieval pointer driven buffer/1  "vi"
  AMA with retrieval pointer driven buffer1/3 -> Terminator3/1
  Constant4/1 -> Divide2/1
  [v] -> Product4/2
  [vintunb] -> Product5/2
  Product2/1 -> Out2/1  "q"
  AMA with retrieval pointer driven buffer5/2 -> Terminator12/1
  AMA with retrieval pointer driven buffer1/1 -> Out8/1, Add/2  "vintbias"

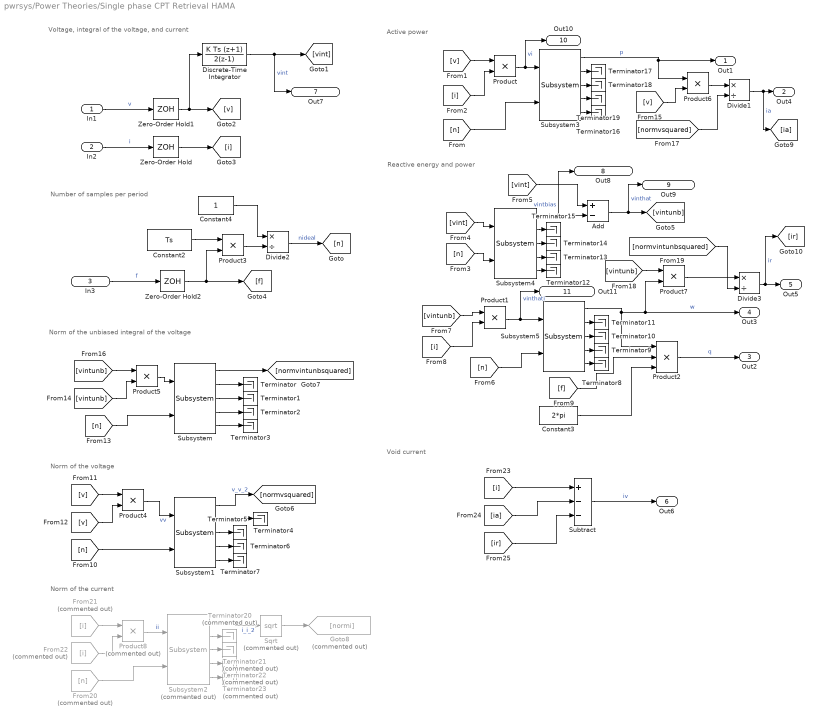
== system pwrsys/Power Theories/Single phase CPT Retrieval HAMA ==
  note: Void current
  note: Number of samples per period
  note: Norm of the voltage
  note: Voltage, integral of the voltage, and current
  note: Reactive energy and power
  note: Active power
  note: Norm of the current
  note: Norm of the unbiased integral of the voltage
  In1 : Inport
  In2 : Inport  Port=2
  In3 : Inport  Port=3
  Add : Sum  Inputs=+-
  Constant2 : Constant  Value=Ts
  Constant3 : Constant  Value=2*pi
  Constant4 : Constant
  Discrete-Time Integrator : DiscreteIntegrator  IntegratorMethod=Integration: Trapezoidal  SampleTime=Ts  ICPrevOutput=DiscIntNeverNeededParam  ICPrevScaledInput=DiscIntNeverNeededParam
  Divide1 : Product  Inputs=*/
  Divide2 : Product  Inputs=*/
  Divide3 : Product  Inputs=*/
  From20 : From  Commented=on  GotoTag=n
  From21 : From  Commented=on  GotoTag=i
  From22 : From  Commented=on  GotoTag=i
  Goto8 : Goto  Commented=on  GotoTag=normi
  Product{,1,3..7} (7 alike) : Product
  Product2 : Product  Inputs=3
  Product8 : Product  Commented=on
  Sqrt : Sqrt  Commented=on  SaturateOnIntegerOverflow=on
  Subsystem{,1,3..5} (5 alike) : $bdroot/Adaptive Moving Averages/Subsystem  NbSize=NbSize  Ts=Ts
  Subsystem2 : $bdroot/Adaptive Moving Averages/Subsystem  Commented=on  NbSize=NbSize  Ts=Ts
  Subtract : Sum  Inputs=+--
  Terminator{,1..19} (20 alike) : Terminator
  Terminator{20..23} (4 alike) : Terminator  Commented=on
  Zero-Order Hold : ZeroOrderHold  SampleTime=Ts
  Zero-Order Hold1 : ZeroOrderHold  SampleTime=Ts
  Zero-Order Hold2 : ZeroOrderHold  SampleTime=Ts
  Out1 : Outport
  Out4 : Outport  Port=2
  Out2 : Outport  Port=3
  Out3 : Outport  Port=4
  Out5 : Outport  Port=5
  Out6 : Outport  Port=6
  Out7 : Outport  Port=7
  Out8 : Outport  Port=8
  Out9 : Outport  Port=9
  Out10 : Outport  Port=10
  Out11 : Outport  Port=11
  wires:
  Product6/1 -> Divide1/1
  [i] -> Product/2
  Product3/1 -> Divide2/2
  Product7/1 -> Divide3/1
  [ia] -> Subtract/2
  [f] -> Product2/2
  Divide3/1 -> [ir], Out5/1  "ir"
  Subsystem2/1 -> Sqrt/1  "i_i_2"
  Product8/1 -> Subsystem2/1  "ii"
  [v] -> Product4/1
  Subtract/1 -> Out6/1  "iv"
  In2/1 -> Zero-Order Hold/1  "i"
  In1/1 -> Zero-Order Hold1/1  "v"
  [v] -> Product/1
  [v] -> Product4/2
  [n] -> Subsystem/2
  [vint] -> Add/1
  Add/1 -> Out9/1, [vintunb]  "vinthat"
  From21/1 -> Product8/1
  Subsystem4/1 -> Out8/1, Add/2  "vintbias"
  Zero-Order Hold2/1 -> Product3/2, [f]
  [ir] -> Subtract/3
  Divide2/1 -> [n]  "nideal"
  Product1/1 -> Subsystem5/1, Out11/1  "vinthati"
  Zero-Order Hold/1 -> [i]
  Divide1/1 -> [ia], Out4/1  "ia"
  [vintunb] -> Product7/1
  Product2/1 -> Out2/1  "q"
  Constant3/1 -> Product2/3
  From22/1 -> Product8/2
  [vintunb] -> Product5/1
  [normvintunbsquared] -> Divide3/2
  Discrete-Time Integrator/1 -> Out7/1, [vint]  "vint"
  [vintunb] -> Product5/2
  [i] -> Subtract/1
  Product5/1 -> Subsystem/1
  [vintunb] -> Product1/1
  Subsystem1/1 -> [normvsquared]  "v_v_2"
  Product/1 -> Subsystem3/1, Out10/1  "vi"
  [v] -> Product6/2
  Constant2/1 -> Product3/1
  [i] -> Product1/2
  Product4/1 -> Subsystem1/1  "vv"
  [n] -> Subsystem1/2
  Subsystem5/1 -> Product2/1, Product7/2, Out3/1  "w"
  [normvsquared] -> Divide1/2
  Zero-Order Hold1/1 -> [v], Discrete-Time Integrator/1
  In3/1 -> Zero-Order Hold2/1  "f"
  Constant4/1 -> Divide2/1
  Subsystem/1 -> [normvintunbsquared]
  Sqrt/1 -> Goto8/1
  Subsystem3/1 -> Product6/1, Out1/1  "p"
  From20/1 -> Subsystem2/2
  [n] -> Subsystem3/2
  [vint] -> Subsystem4/1
  [n] -> Subsystem4/2
  [n] -> Subsystem5/2
  Subsystem/2 -> Terminator/1
  Subsystem/3 -> Terminator1/1
  Subsystem/4 -> Terminator2/1
  Subsystem/5 -> Terminator3/1
  Subsystem1/2 -> Terminator4/1
  Subsystem1/3 -> Terminator5/1
  Subsystem1/4 -> Terminator6/1
  Subsystem1/5 -> Terminator7/1
  Subsystem5/5 -> Terminator8/1
  Subsystem5/4 -> Terminator9/1
  Subsystem5/3 -> Terminator10/1
  Subsystem5/2 -> Terminator11/1
  Subsystem4/5 -> Terminator12/1
  Subsystem4/4 -> Terminator13/1
  Subsystem4/3 -> Terminator14/1
  Subsystem4/2 -> Terminator15/1
  Subsystem3/5 -> Terminator16/1
  Subsystem3/2 -> Terminator17/1
  Subsystem3/3 -> Terminator18/1
  Subsystem3/4 -> Terminator19/1
  Subsystem2/2 -> Terminator20/1
  Subsystem2/3 -> Terminator21/1
  Subsystem2/4 -> Terminator22/1
  Subsystem2/5 -> Terminator23/1

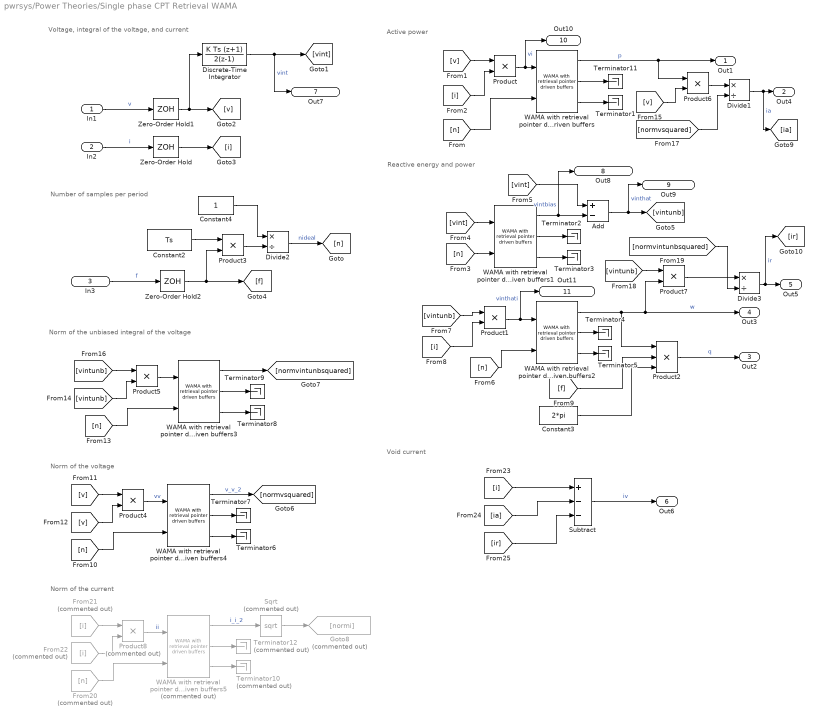
== system pwrsys/Power Theories/Single phase CPT Retrieval WAMA ==
  note: Voltage, integral of the voltage, and current
  note: Number of samples per period
  note: Reactive energy and power
  note: Active power
  note: Norm of the voltage
  note: Norm of the unbiased integral of the voltage
  note: Norm of the current
  note: Void current
  In1 : Inport
  In2 : Inport  Port=2
  In3 : Inport  Port=3
  Add : Sum  Inputs=+-
  Constant2 : Constant  Value=Ts
  Constant3 : Constant  Value=2*pi
  Constant4 : Constant
  Discrete-Time Integrator : DiscreteIntegrator  IntegratorMethod=Integration: Trapezoidal  SampleTime=Ts  ICPrevOutput=DiscIntNeverNeededParam  ICPrevScaledInput=DiscIntNeverNeededParam
  Divide1 : Product  Inputs=*/
  Divide2 : Product  Inputs=*/
  Divide3 : Product  Inputs=*/
  From20 : From  Commented=on  GotoTag=n
  From21 : From  Commented=on  GotoTag=i
  From22 : From  Commented=on  GotoTag=i
  Goto8 : Goto  Commented=on  GotoTag=normi
  Product{,1,3..7} (7 alike) : Product
  Product2 : Product  Inputs=3
  Product8 : Product  Commented=on
  Sqrt : Sqrt  Commented=on  SaturateOnIntegerOverflow=on
  Subtract : Sum  Inputs=+--
  Terminator{1..9,11} (10 alike) : Terminator
  Terminator10 : Terminator  Commented=on
  Terminator12 : Terminator  Commented=on
  WAMA with retrieval pointer driven buffers{,1..4} (5 alike) : $bdroot/Adaptive Moving Averages/WAMA with retrieval pointer driven buffers  NbSize=NbSize  Ts=Ts
  WAMA with retrieval pointer driven buffers5 : $bdroot/Adaptive Moving Averages/WAMA with retrieval pointer driven buffers  Commented=on  NbSize=NbSize  Ts=Ts
  Zero-Order Hold : ZeroOrderHold  SampleTime=Ts
  Zero-Order Hold1 : ZeroOrderHold  SampleTime=Ts
  Zero-Order Hold2 : ZeroOrderHold  SampleTime=Ts
  Out1 : Outport
  Out4 : Outport  Port=2
  Out2 : Outport  Port=3
  Out3 : Outport  Port=4
  Out5 : Outport  Port=5
  Out6 : Outport  Port=6
  Out7 : Outport  Port=7
  Out8 : Outport  Port=8
  Out9 : Outport  Port=9
  Out10 : Outport  Port=10
  Out11 : Outport  Port=11
  wires:
  Discrete-Time Integrator/1 -> Out7/1, [vint]  "vint"
  In3/1 -> Zero-Order Hold2/1  "f"
  Zero-Order Hold1/1 -> [v], Discrete-Time Integrator/1
  [i] -> Subtract/1
  WAMA with retrieval pointer driven buffers3/1 -> [normvintunbsquared]
  Product5/1 -> WAMA with retrieval pointer driven buffers3/1
  WAMA with retrieval pointer driven buffers3/2 -> Terminator9/1
  WAMA with retrieval pointer driven buffers3/3 -> Terminator8/1
  Product4/1 -> WAMA with retrieval pointer driven buffers4/1  "vv"
  WAMA with retrieval pointer driven buffers4/3 -> Terminator6/1
  WAMA with retrieval pointer driven buffers4/2 -> Terminator7/1
  WAMA with retrieval pointer driven buffers4/1 -> [normvsquared]  "v_v_2"
  [n] -> WAMA with retrieval pointer driven buffers4/2
  [vint] -> WAMA with retrieval pointer driven buffers1/1
  WAMA with retrieval pointer driven buffers5/3 -> Terminator10/1
  WAMA with retrieval pointer driven buffers1/2 -> Terminator2/1
  WAMA with retrieval pointer driven buffers/2 -> Terminator11/1
  WAMA with retrieval pointer driven buffers/3 -> Terminator1/1
  WAMA with retrieval pointer driven buffers2/2 -> Terminator4/1
  Product1/1 -> Out11/1, WAMA with retrieval pointer driven buffers2/1  "vinthati"
  [v] -> Product6/2
  WAMA with retrieval pointer driven buffers2/1 -> Product7/2, Out3/1, Product2/1  "w"
  Product/1 -> Out10/1, WAMA with retrieval pointer driven buffers/1  "vi"
  [vintunb] -> Product7/1
  [normvsquared] -> Divide1/2
  [normvintunbsquared] -> Divide3/2
  Divide1/1 -> [ia], Out4/1  "ia"
  Zero-Order Hold/1 -> [i]
  [vint] -> Add/1
  Constant3/1 -> Product2/3
  [i] -> Product1/2
  [vintunb] -> Product1/1
  Constant2/1 -> Product3/1
  [vintunb] -> Product5/1
  [ir] -> Subtract/3
  From22/1 -> Product8/2
  [n] -> WAMA with retrieval pointer driven buffers2/2
  WAMA with retrieval pointer driven buffers5/2 -> Terminator12/1
  Zero-Order Hold2/1 -> Product3/2, [f]
  Product7/1 -> Divide3/1
  WAMA with retrieval pointer driven buffers1/3 -> Terminator3/1
  Sqrt/1 -> Goto8/1
  Divide2/1 -> [n]  "nideal"
  WAMA with retrieval pointer driven buffers5/1 -> Sqrt/1  "i_i_2"
  Constant4/1 -> Divide2/1
  Product2/1 -> Out2/1  "q"
  [n] -> WAMA with retrieval pointer driven buffers3/2
  Product3/1 -> Divide2/2
  [n] -> WAMA with retrieval pointer driven buffers/2
  From20/1 -> WAMA with retrieval pointer driven buffers5/2
  [vintunb] -> Product5/2
  [v] -> Product4/2
  Product8/1 -> WAMA with retrieval pointer driven buffers5/1  "ii"
  Product6/1 -> Divide1/1
  WAMA with retrieval pointer driven buffers1/1 -> Out8/1, Add/2  "vintbias"
  Add/1 -> Out9/1, [vintunb]  "vinthat"
  [f] -> Product2/2
  In1/1 -> Zero-Order Hold1/1  "v"
  From21/1 -> Product8/1
  WAMA with retrieval pointer driven buffers/1 -> Product6/1, Out1/1  "p"
  Subtract/1 -> Out6/1  "iv"
  [i] -> Product/2
  In2/1 -> Zero-Order Hold/1  "i"
  [n] -> WAMA with retrieval pointer driven buffers1/2
  Divide3/1 -> [ir], Out5/1  "ir"
  [v] -> Product4/1
  WAMA with retrieval pointer driven buffers2/3 -> Terminator5/1
  [v] -> Product/1
  [ia] -> Subtract/2

== system pwrsys/Transformations/abc to xyz ==
  note: Clark Transform
  abc : Inport
  Demux : Demux  Outputs=3
  Gain : Gain  Gain=c
  Gain1 : Gain  Gain=a
  Gain2 : Gain  Gain=b
  Gain4 : Gain  Gain=2
  Mux : Mux  Inputs=3
  Sum1 : Sum  Inputs=+-
  Sum2 : Sum  Inputs=+++
  Sum3 : Sum  Inputs=+--
  xyz : Outport
  wires:
  abc/1 -> Demux/1
  Demux/1 -> Sum2/1, Gain4/1  "a"
  Gain/1 -> Mux/3  "z"
  Gain2/1 -> Mux/2  "y"
  Gain1/1 -> Mux/1  "x"
  Mux/1 -> xyz/1
  Gain4/1 -> Sum3/1
  Demux/2 -> Sum2/2, Sum1/1, Sum3/2  "b"
  Demux/3 -> Sum2/3, Sum1/2, Sum3/3  "c"
  Sum3/1 -> Gain1/1  "B"
  Sum1/1 -> Gain2/1
  Sum2/1 -> Gain/1

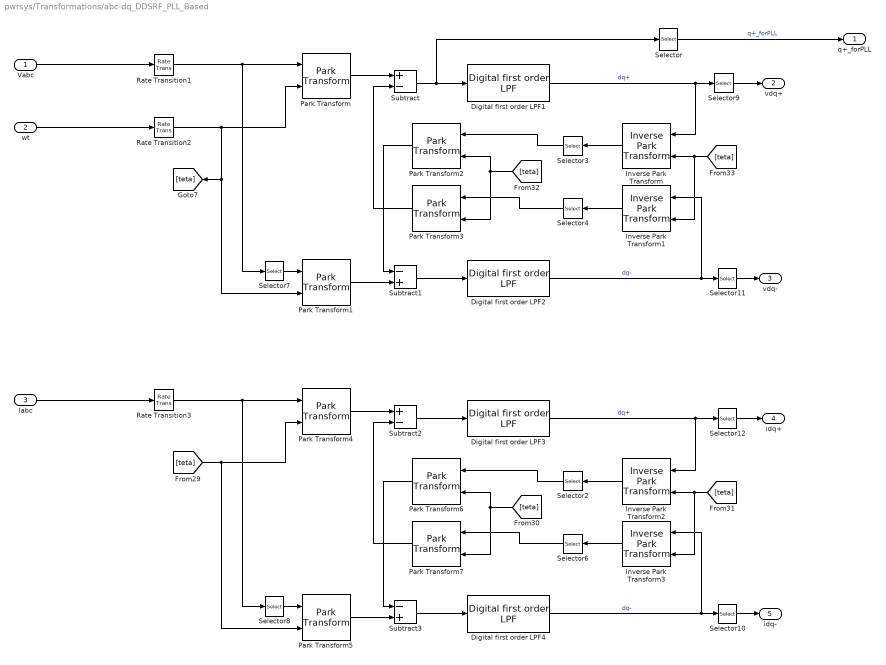
== system pwrsys/Transformations/abc-dq_DDSRF_PLL_Based ==
  Vabc : Inport
  wt : Inport  Port=2
  Iabc : Inport  Port=3
  Digital first order LPF{1..4} (4 alike) : $bdroot/Basic Blocks/Digital first order LPF  Ts=Ts  fcutout=fc
  Inverse Park Transform{,1..3} (4 alike) : peTransforms/Inverse Park Transform  AxisAlignment=Q-axis  PowerInvariant=off
  Park Transform{,1..7} (8 alike) : peTransforms/Park Transform  AxisAlignment=Q-axis  PowerInvariant=off
  Rate Transition1 : RateTransition  OutPortSampleTime=Ts
  Rate Transition2 : RateTransition  OutPortSampleTime=Ts
  Rate Transition3 : RateTransition  OutPortSampleTime=Ts
  Selector : Selector  InputPortWidth=3  IndexOptions=Index vector (dialog)  Indices=2  OutputSizes=1
  Selector{9..12} (4 alike) : Selector  InputPortWidth=3  IndexOptions=Index vector (dialog)  Indices=[1 2]  OutputSizes=1
  Selector{2..4,6..8} (6 alike) : Selector  InputPortWidth=3  IndexOptions=Index vector (dialog)  Indices=[1 3 2]  OutputSizes=1
  Subtract : Sum  Inputs=+-
  Subtract1 : Sum  Inputs=-+
  Subtract2 : Sum  Inputs=+-
  Subtract3 : Sum  Inputs=-+
  q+_forPLL : Outport
  vdq+ : Outport  Port=2
  vdq- : Outport  Port=3
  idq+ : Outport  Port=4
  idq- : Outport  Port=5
  wires:
  Selector/1 -> q+_forPLL/1  "q+_forPLL"
  [teta] -> Inverse Park Transform2/2, Inverse Park Transform3/2
  Rate Transition3/1 -> Selector8/1, Park Transform4/1
  Selector11/1 -> vdq-/1
  Rate Transition1/1 -> Selector7/1, Park Transform/1
  Digital first order LPF4/1 -> Inverse Park Transform3/1, Selector10/1  "dq-"
  Inverse Park Transform3/1 -> Selector6/1
  Rate Transition2/1 -> [teta], Park Transform1/2, Park Transform/2
  Selector4/1 -> Park Transform3/1
  Iabc/1 -> Rate Transition3/1
  [teta] -> Park Transform6/2, Park Transform7/2
  Subtract2/1 -> Digital first order LPF3/1
  Park Transform1/1 -> Subtract1/2
  Selector6/1 -> Park Transform7/1
  Selector8/1 -> Park Transform5/1
  Park Transform7/1 -> Subtract2/2
  Digital first order LPF2/1 -> Selector11/1, Inverse Park Transform1/1  "dq-"
  Selector9/1 -> vdq+/1
  Inverse Park Transform1/1 -> Selector4/1
  Inverse Park Transform2/1 -> Selector2/1
  [teta] -> Park Transform2/2, Park Transform3/2
  Selector10/1 -> idq-/1
  Park Transform2/1 -> Subtract1/1
  Selector2/1 -> Park Transform6/1
  Park Transform5/1 -> Subtract3/2
  Subtract3/1 -> Digital first order LPF4/1
  Subtract1/1 -> Digital first order LPF2/1
  Park Transform/1 -> Subtract/1
  Digital first order LPF3/1 -> Inverse Park Transform2/1, Selector12/1  "dq+"
  Selector12/1 -> idq+/1
  Selector3/1 -> Park Transform2/1
  wt/1 -> Rate Transition2/1
  Park Transform6/1 -> Subtract3/1
  [teta] -> Park Transform5/2, Park Transform4/2
  Park Transform4/1 -> Subtract2/1
  Subtract/1 -> Digital first order LPF1/1, Selector/1
  [teta] -> Inverse Park Transform/2, Inverse Park Transform1/2
  Digital first order LPF1/1 -> Selector9/1, Inverse Park Transform/1  "dq+"
  Vabc/1 -> Rate Transition1/1
  Selector7/1 -> Park Transform1/1
  Inverse Park Transform/1 -> Selector3/1
  Park Transform3/1 -> Subtract/2
